simulink model "phase2_Q2"  (R2022b)
settings: Solver=ode4  StartTime=0.0  StopTime=15  FixedStep=0.01  RelTol=1e-3
InitFcn:
  | state_space
StopFcn:
  | ending
values from neighbouring files (symbols this model uses):
  g = 9.81    [initial.m]
  Initial_Conditions = [chi0.x;chi0.y;chi0.z ... (first row only)    [initial.m]
undefined symbols (not defined in the file or in its folder): A, B, body, C, D, RRV
settings Model: Creator=User  LastModifiedBy=Alire

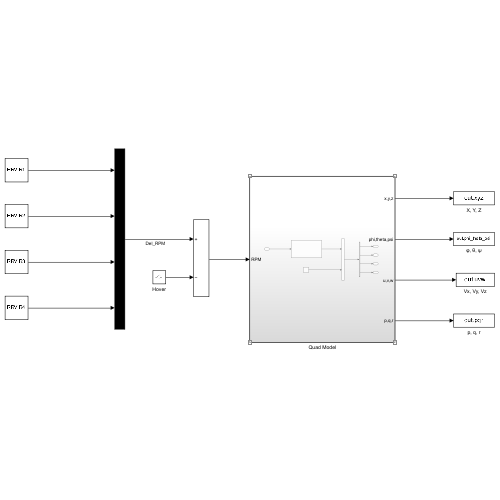
[thumbnail: Simulink's stored preview of the top-level diagram]
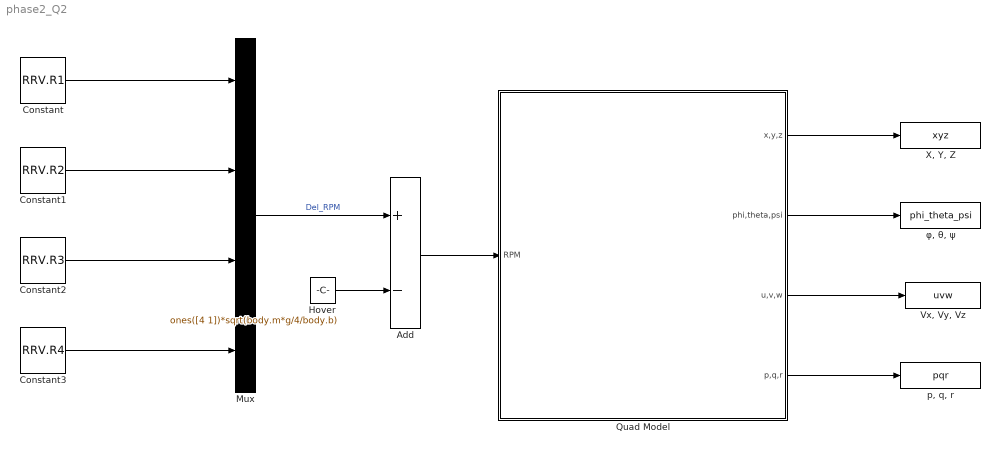
== system phase2_Q2 ==
  Add : Sum  Inputs=+-
  Constant : Constant  Value=RRV.R1
  Constant1 : Constant  Value=RRV.R2
  Constant2 : Constant  Value=RRV.R3
  Constant3 : Constant  Value=RRV.R4
  Hover : Constant  Value=ones([4 1])*sqrt(body.m*g/4/body.b)
  Mux : Mux
  Quad Model : Subsystem
  "Vx, Vy, Vz" : ToWorkspace  VariableName=uvw  SampleTime=-1
  "X, Y, Z" : ToWorkspace  VariableName=xyz  SampleTime=-1
  "p, q, r" : ToWorkspace  VariableName=pqr  SampleTime=-1
  "φ, θ, ψ" : ToWorkspace  VariableName=phi_theta_psi  SampleTime=-1
  wires:
  Constant1/1 -> Mux/2
  Constant3/1 -> Mux/4
  Constant/1 -> Mux/1
  Constant2/1 -> Mux/3
  Quad Model/1(x,y,z) -> "X, Y, Z"/1
  Mux/1 -> Add/1  "Del_RPM"
  Quad Model/3(u,v,w) -> "Vx, Vy, Vz"/1
  Quad Model/4(p,q,r) -> "p, q, r"/1
  Quad Model/2(phi,theta,psi) -> "φ, θ, ψ"/1
  Hover/1 -> Add/2
  Add/1 -> Quad Model/1(RPM)

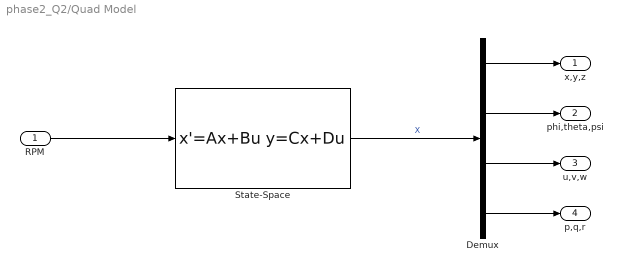
== system phase2_Q2/Quad Model ==
  RPM : Inport
  Demux : Demux
  State-Space : StateSpace  A=A  B=B  C=C  D=D  InitialCondition=Initial_Conditions  ParameterTunability=Optimized
  x,y,z : Outport
  phi,theta,psi : Outport  Port=2
  u,v,w : Outport  Port=3
  p,q,r : Outport  Port=4
  wires:
  Demux/1 -> x,y,z/1
  Demux/2 -> phi,theta,psi/1
  Demux/3 -> u,v,w/1
  Demux/4 -> p,q,r/1
  RPM/1 -> State-Space/1
  State-Space/1 -> Demux/1  "X"
